simulink model "multiply_rounding_example"  (R2019b)
settings: Solver=FixedStepDiscrete  StartTime=0.0  StopTime=1000  RelTol=1e-3
PostLoadFcn:
  | InputWL1 = 16;
  | InputFL1 = 15;
  | 
  | InputWL2 = 24;
  | InputFL2 = 23;
  | 
  | OutputWL = 24;
InitFcn:
  | % Full-precision mult DT
  | MultWL = InputWL1 + InputWL2;
  | MultFL = InputFL1 + InputFL2;
  | IntBits = MultWL - MultFL; % integer bits
  | 
  | % Mult DT after rounding
  | OutputFL = OutputWL - IntBits;
libraries: simulink x2
settings Model: DataTypeOverride=Off  Creator=cchung  LastModifiedBy=cchung
settings OptimizationCC: BlockReduction=off  ConditionallyExecuteInputs=off  DefaultParameterBehavior=Inlined
settings DebuggingCC: AlgebraicLoopMsg=error  SingleTaskRateTransMsg=error
settings HardwareCC: ProdBitPerPointer=32  ProdBitPerSizeT=32  ProdBitPerPtrDiffT=32  ProdLargestAtomicFloat=None  ProdIntDivRoundTo=Undefined  ProdEndianess=Unspecified  ProdWordSize=32  ProdHWDeviceType=ASIC/FPGA->ASIC/FPGA  TargetBitPerPointer=64  TargetBitPerSizeT=64  TargetBitPerPtrDiffT=64  TargetLongLongMode=on  TargetIntDivRoundTo=Zero  TargetEndianess=LittleEndian  TargetWordSize=64  TargetHWDeviceType=Custom Processor->MATLAB Host Computer  ProdEqTarget=off

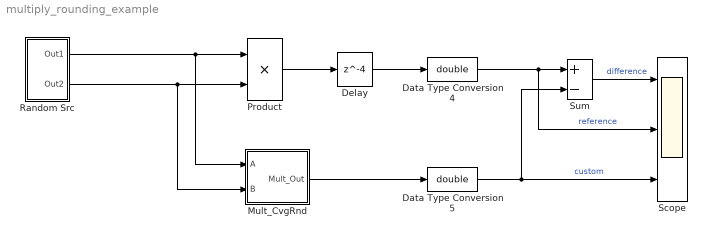
== system multiply_rounding_example ==
  Data Type Conversion4 : DataTypeConversion  OutDataTypeStr=double
  Data Type Conversion5 : DataTypeConversion  OutDataTypeStr=double
  Delay : Delay  DelayLength=4
  Mult_CvgRnd : Subsystem
  Product : Product  OutDataTypeStr=fixdt(1,OutputWL,OutputFL)  RndMeth=Convergent
  Random Src : Subsystem
  Scope : Scope  NumInputPorts=3
  Sum : Sum  Inputs=+-
  wires:
  Product/1 -> Delay/1
  Delay/1 -> Data Type Conversion4/1
  Mult_CvgRnd/1(Mult_Out) -> Data Type Conversion5/1
  Data Type Conversion4/1 -> Sum/1, Scope/2  "reference"
  Data Type Conversion5/1 -> Scope/3, Sum/2  "custom"
  Sum/1 -> Scope/1  "difference"
  Random Src/2(Out2) -> Mult_CvgRnd/2(B), Product/2
  Random Src/1(Out1) -> Mult_CvgRnd/1(A), Product/1

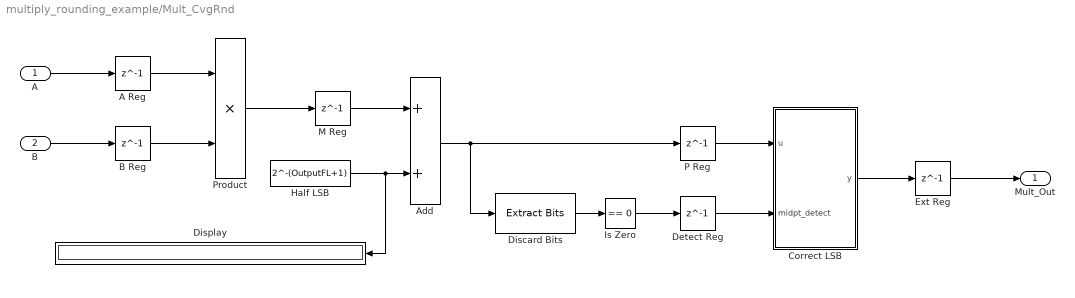
== system multiply_rounding_example/Mult_CvgRnd ==
  A : Inport
  B : Inport  Port=2
  A Reg : Delay  DelayLength=1
      settings: AttributesFormatString=ResetType : none
  Add : Sum  OutDataTypeStr=Inherit: Same as first input
  B Reg : Delay  DelayLength=1
      settings: AttributesFormatString=ResetType : none
  Correct LSB : MATLAB Function  TreatAsAtomicUnit=on
  Detect Reg : Delay  DelayLength=1
      settings: AttributesFormatString=ResetType : none
  Discard Bits : simulink/Logic and Bit Operations/Extract Bits  bitsToExtract=Range ending with least significant bit  numBits=MultWL-OutputWL  bitIdxRange=[0 7]  outScalingMode=Treat bit field as an integer
  Display : Display
      settings: Format=binary (Stored Integer)
  Ext Reg : Delay  DelayLength=1
      settings: AttributesFormatString=ResetType : none
  Half LSB : Constant  Value=2^-(OutputFL+1)  OutDataTypeStr=Inherit: Inherit via back propagation  SampleTime=-1
  Is Zero : simulink/Logic and Bit Operations/Compare To Constant  relop===  const=0  OutDataTypeStr=boolean
  M Reg : Delay  DelayLength=1
      settings: AttributesFormatString=ResetType : none
  P Reg : Delay  DelayLength=1
      settings: AttributesFormatString=ResetType : none
  Product : Product
  Mult_Out : Outport
  wires:
  Product/1 -> M Reg/1
  A/1 -> A Reg/1
  B/1 -> B Reg/1
  A Reg/1 -> Product/1
  B Reg/1 -> Product/2
  Half LSB/1 -> Display/1, Add/2
  M Reg/1 -> Add/1
  Add/1 -> Discard Bits/1, P Reg/1
  Discard Bits/1 -> Is Zero/1
  P Reg/1 -> Correct LSB/1(u)
  Detect Reg/1 -> Correct LSB/2(midpt_detect)
  Ext Reg/1 -> Mult_Out/1
  Correct LSB/1(y) -> Ext Reg/1
  Is Zero/1 -> Detect Reg/1

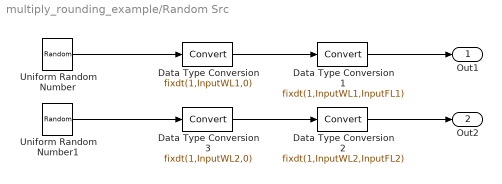
== system multiply_rounding_example/Random Src ==
  Data Type Conversion : DataTypeConversion  OutDataTypeStr=fixdt(1,InputWL1,0)
  Data Type Conversion1 : DataTypeConversion  OutDataTypeStr=fixdt(1,InputWL1,InputFL1)  ConvertRealWorld=Stored Integer (SI)
  Data Type Conversion2 : DataTypeConversion  OutDataTypeStr=fixdt(1,InputWL2,InputFL2)  ConvertRealWorld=Stored Integer (SI)
  Data Type Conversion3 : DataTypeConversion  OutDataTypeStr=fixdt(1,InputWL2,0)
  Uniform Random Number : UniformRandomNumber  Minimum=-2^(InputWL1-1)  Maximum=2^(InputWL1-1)-1  Seed=randi([0 10])  SampleTime=1
  Uniform Random Number1 : UniformRandomNumber  Minimum=-2^(InputWL2-1)  Maximum=2^(InputWL2-1)-1  Seed=randi([0 10])  SampleTime=1
  Out1 : Outport
  Out2 : Outport  Port=2
  wires:
  Data Type Conversion3/1 -> Data Type Conversion2/1
  Data Type Conversion/1 -> Data Type Conversion1/1
  Data Type Conversion1/1 -> Out1/1
  Data Type Conversion2/1 -> Out2/1
  Uniform Random Number/1 -> Data Type Conversion/1
  Uniform Random Number1/1 -> Data Type Conversion3/1

== matlab function multiply_rounding_example/Mult_CvgRnd/Correct LSB ==
  settings: fimath=hdlfimath
  data: u input; y output; midpt_detect input; OutputWL parameter; OutputFL parameter
function y = fcn(u,midpt_detect,OutputWL, OutputFL)
%#codegen

NewLSB = u.WordLength - OutputWL + 1;
OutputDT = numerictype(1,OutputWL,OutputFL);

if midpt_detect
    % Round mid-point to even
    x = bitconcat(bitsliceget(u,u.WordLength,NewLSB+1),fi(0,0,1,0));
else
    x = bitsliceget(u,u.WordLength,NewLSB);
end

y = reinterpretcast(x,OutputDT);
